simulink model "Converter_2"  (R2018a)
settings: Solver=ode45  StartTime=0.0  StopTime=3  FixedStep=Ts  RelTol=1e-3
InitFcn:
  | load('initial_C2.mat')
  | Ts=5e-4;
  | Ts_Power=Ts;
  | Ts_Control=Ts;
  | 
  | 
  | P_order = 0.9; %refrence power
  | V_order = .9965; %refrence voltage
  | Q_order = 0.4;
  | w_order = 1;
  | 
  | step_P_order = 2; %Step p_order at 5 sec.
  | 
  | %% DROOP COFFEICIENT
  | Kpf = 5; % Kpf = 1/m.
  | n = .1;
  | 
  | 
  | Kp = 0.3; Ki =5; % inner loop
  | %Outer loop
  | Kpp =1; Kip =100;
  | Kpv =.5; Kiv =50;
  | %Kpv =0.40; Kiv =40;
  | 
  | Kp_PLL = 60; Ki_PLL = 1400; % PLL 13 Hz
  | 
  | 
  | Cs = 0.25; % Shunt capacitor in pu
  | 
  | 
  | 
  | wb=2*pi*60;
  | Sb=10e3;
  | Vb=260;
  | Vconv=260;
  | Zb=Vb^2/Sb;
  | 
  | X=0.15;
  | 
  | %% Tirp Transmision line
  | Tstep3=5; % trip line: Xg_start-->Xg_mid
  | Tstep2=7; % trip line: Xg_mid-->Xg_final
  | 
  | 
  | 
  | Xg_start=1.172; Xg_mid=1.73; Xg_final=1.174;
  | %Xg_start=0.765; Xg_mid=0.95; Xg_final=1.08;
  | 
  | 
  | Xgpu2=Xg_mid*Xg_final/(Xg_final-Xg_mid);
  | Xgpu3=Xg_start*(Xg_final*Xgpu2)/(Xg_final*Xgpu2-Xg_start*(Xg_final+Xgpu2));
  | 
  | %Line 1
  | Xgpu1=Xg_final;
  | Rgpu1=0.1*Xgpu1;%Rg=0.1*Xg;
  | Xg1=Xgpu1*Zb;
  | Lg1=Xg1/wb;   %H
  | Rg1=Rgpu1*Zb; %ohm
  | %Line 2
  | Rgpu2=0.1*Xgpu2;%Rg=0.1*Xg;
  | Xg2=Xgpu2*Zb;
  | Lg2=Xg2/wb;   %H
  | Rg2=Rgpu2*Zb; %ohm
  | %Line 3
  | Rgpu3=0.1*Xgpu3;%Rg=0.1*Xg;
  | Xg3=Xgpu3*Zb;
  | Lg3=Xg3/wb;   %H
  | Rg3=Rgpu3*Zb; %ohm
undefined symbols (not defined in the file or in its folder): DiscIntNeverNeededParam
libraries: powerlib x14, powerlib_meascontrol x5, simulink x3
Description:
  | Copyright 2008-2017 The MathWorks, Inc.
settings Model: Creator=MathWorks  LastModifiedBy=almut
settings DataIOCC: FinalStateName=Sup_PLL2a  InitialState=Sup_PLL2a  LimitDataPoints=on  LoadInitialState=on  SaveFormat=Array  SignalLoggingSaveFormat=ModelDataLogs
settings OptimizationCC: ExpressionDepthLimit=2147483647  EfficientMapNaN2IntZero=off  LifeSpan=inf
settings DebuggingCC: UnderspecifiedInitializationDetection=Classic  MergeDetectMultiDrivingBlocksExec=none  SolverPrmCheckMsg=warning  FcnCallInpInsideContextMsg=warning  StateNameClashWarn=warning  SFUnexpectedBacktrackingDiag=warning  SFNoUnconditionalDefaultTransitionDiag=warning  SFExecutionAtInitializationDiag=none
settings HardwareCC: ProdBitPerPointer=32  ProdBitPerSizeT=32  ProdBitPerPtrDiffT=32  ProdLargestAtomicFloat=None  ProdIntDivRoundTo=Undefined  ProdEndianess=Unspecified  ProdWordSize=32  ProdHWDeviceType=32-bit Generic  TargetBitPerPointer=64  TargetBitPerSizeT=64  TargetBitPerPtrDiffT=64  TargetLongLongMode=on  TargetIntDivRoundTo=Zero  TargetEndianess=LittleEndian  TargetWordSize=64  TargetHWDeviceType=MATLAB Host  ProdEqTarget=off
settings ModelReferenceCC: PropagateSignalLabelsOutOfModel=off
settings CodeAppCC: MaxIdLength=128  StateflowObjectComments=on
settings GRTTargetCC: TargetLangStandard=C89/C90 (ANSI)  CombineOutputUpdateFcns=off  GRTInterface=on
settings ConfigComp: CovMetricSettings=dw  CovHtmlReporting=on  CovSaveCumulativeToWorkspaceVar=on  CovSaveSingleToWorkspaceVar=on  CovExternalEMLEnable=off  CovSFcnEnable=off
settings SimscapeCC: SimscapeNormalizeSystem=off

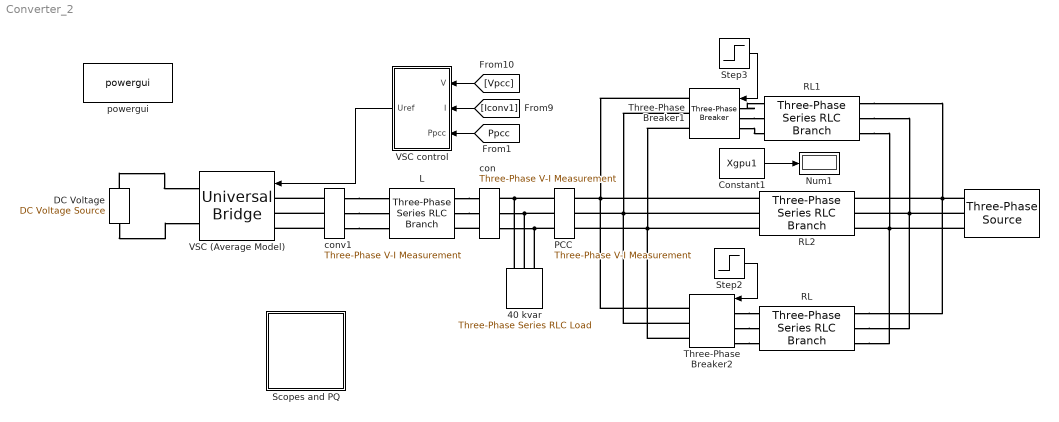
== system Converter_2 ==
  " " : powerlib/Electrical Sources/Three-Phase Source  InternalConnection=Yg  VoltagePhases=off  Voltage=260  PhaseAngle=0  Voltage_phases=[25e3 25e3 25e3]/sqrt(3)  PhaseAngles_phases=[0 -120 +120]  Frequency=60  NonIdealSource=off  SpecifyImpedance=on  Resistance=0.8929  Inductance=16.58e-3  ShortCircuitLevel=2500e6  BaseVoltage=120e3  XRratio=7  BusType=swing  Pref=0  Qref=0  Prefabc=[10e3, 10e3, 10e3]  Qrefabc=[0, 0, 0]  Qmin=-inf  Qmax=inf
  40 kvar : powerlib/Elements/Three-Phase Series RLC Load  LConnTagsString=A|B|C  Configuration=Y (grounded)  NominalVoltage=260  Vabc=[1e3 1e3 1e3]  Vabcp=[1e3 1e3 1e3]  NominalFrequency=60  UnbalancedPower=off  ActivePower=0  InductivePower=0  CapacitivePower=10e3*0.25  Pabc=[10e3 9e3 11e3]  QLabc=[100 90 110]  QCabc=[100 90 110]  Pabcp=[10e3 9e3 11e3]  QLabcp=[100 90 110]  QCabcp=[100 90 110]  Measurements=None  LoadType=constant Z
  Constant1 : Constant  Value=Xgpu1
  "DC Voltage " : powerlib/Electrical Sources/DC Voltage Source  Amplitude=500  Measurements=None
  L : powerlib/Elements/Three-Phase Series RLC Branch  LConnTagsString=A|B|C  RConnTagsString=A|B|C  BranchType=RL  Resistance=X/50*260^2/10e3  Inductance=X/(2*pi*60)*260^2/10e3  Capacitance=inf  Measurements=None
  Num1 : Display
  PCC : powerlib/Measurements/Three-Phase V-I Measurement  VoltageMeasurement=phase-to-ground  SetLabelV=on  LabelV=Vpcc  Vpu=on  VpuLL=off  CurrentMeasurement=yes  SetLabelI=on  LabelI=Ipcc  Ipu=on  Pbase=10e3  Vbase=260  OutputType=Magnitude  PhasorSimulation=off  PSBequivalent=0
  RL : powerlib/Elements/Three-Phase Series RLC Branch  LConnTagsString=A|B|C  RConnTagsString=A|B|C  BranchType=RL  Resistance=Rg2  Inductance=Lg2  Capacitance=[]  Measurements=None
  RL1 : powerlib/Elements/Three-Phase Series RLC Branch  LConnTagsString=A|B|C  RConnTagsString=A|B|C  BranchType=RL  Resistance=Rg3  Inductance=Lg3  Capacitance=[]  Measurements=None
  RL2 : powerlib/Elements/Three-Phase Series RLC Branch  LConnTagsString=A|B|C  RConnTagsString=A|B|C  BranchType=RL  Resistance=Rg1  Inductance=Lg1  Capacitance=[]  Measurements=None
  "Scopes and PQ " : Subsystem
  Step2 : Step  Time=Tstep2  Before=1  After=0  SampleTime=0
  Step3 : Step  Time=Tstep3  Before=1  After=0  SampleTime=0
  Three-Phase Breaker1 : powerlib/Elements/Three-Phase Breaker  InitialState=closed  SwitchA=on  SwitchB=on  SwitchC=on  SwitchTimes=[1 1000]  External=on  BreakerResistance=0.001  SnubberResistance=1e6  SnubberCapacitance=inf  Measurements=None
  Three-Phase Breaker2 : powerlib/Elements/Three-Phase Breaker  InitialState=closed  SwitchA=on  SwitchB=on  SwitchC=on  SwitchTimes=[1 1000]  External=on  BreakerResistance=0.001  SnubberResistance=1e6  SnubberCapacitance=inf  Measurements=None
  VSC (Average Model) : powerlib/Power Electronics/Universal Bridge  Arms=3  SnubberResistance=1e5  SnubberCapacitance=inf  Device=Average-model based VSC  Ron=1e-3  Lon=0  ForwardVoltages="[  0  0  ]"  ForwardVoltage=0  GTOparameters=[ 10e-6 , 20e-6 ]  IGBTparameters=[ 1e-6 , 2e-6 ]  Measurements=None  Measurements_2=None  converterType=Rectifier
  VSC control : Subsystem
  con : powerlib/Measurements/Three-Phase V-I Measurement  VoltageMeasurement=phase-to-ground  SetLabelV=on  LabelV=Vcon  Vpu=on  VpuLL=off  CurrentMeasurement=yes  SetLabelI=on  LabelI=Icon  Ipu=on  Pbase=10e3  Vbase=260  OutputType=Magnitude  PhasorSimulation=off  PSBequivalent=0
  conv1 : powerlib/Measurements/Three-Phase V-I Measurement  VoltageMeasurement=phase-to-ground  SetLabelV=on  LabelV=Vconv1  Vpu=on  VpuLL=off  CurrentMeasurement=yes  SetLabelI=on  LabelI=Iconv1  Ipu=on  Pbase=10e3  Vbase=260  OutputType=Magnitude  PhasorSimulation=off  PSBequivalent=0
  powergui : powerlib/powergui  Priority=1  SimulationMode=Discrete  SampleTime=Ts  frequency=60  Iterations=50  frequencyindice=0  Pbase=100e6  ErrMax=1e-4  UnitsV=kV  UnitsW=MW  buscounter=0  FunctionMessages=off  echomessages=off  EnableUseOfTLC=off  CurrentSourceSwitches=off  DisableSnubberDevices=off  DisableRonSwitches=off  DisableVfSwitches=off  DisplayEquations=off  SolverType=Tustin/Backward Euler (TBE)  Interpol=off  ExternalGateDelay=off  methode=off  Ts=100  x0status=blocks  SPID=off  SwTol=0  HookPort=off  RestoreLinks=warning  ResistiveCurrentMeasurement=off  Frange=[0:2:500]  Ylog=off  Xlog=on  ShowGrid=off  save=off  variable=ZData  structure=y  ZoomFFT=off  StartTime=2.5  cycles=30  DisplayStyle=2  fundamental=60  FreqAxis=off  MaxFrequency=100  frequencyindicesteady=1  RmsSteady=1  display=off
  wires:
  VSC control/1(Uref) -> VSC (Average Model)/1
  [Vpcc] -> VSC control/1(V)
  [Iconv1] -> VSC control/2(I)
  Step2/1 -> Three-Phase Breaker2/1
  Constant1/1 -> Num1/1
  Step3/1 -> Three-Phase Breaker1/1
  [Ppcc] -> VSC control/3(Ppcc)
  connections:
  con/LConn3 -- L/RConn3
  L/RConn1 -- con/LConn1
  L/RConn2 -- con/LConn2
  PCC/LConn1 -- 40 kvar/LConn1 -- con/RConn1
  con/RConn3 -- 40 kvar/LConn3 -- PCC/LConn3
  con/RConn2 -- 40 kvar/LConn2 -- PCC/LConn2
  conv1/RConn1 -- L/LConn1
  conv1/RConn3 -- L/LConn3
  conv1/RConn2 -- L/LConn2
  conv1/LConn1 -- VSC (Average Model)/LConn1
  conv1/LConn2 -- VSC (Average Model)/LConn2
  conv1/LConn3 -- VSC (Average Model)/LConn3
  "DC Voltage "/RConn1 -- VSC (Average Model)/RConn1
  "DC Voltage "/LConn1 -- VSC (Average Model)/RConn2
  Three-Phase Breaker2/LConn3 -- RL/RConn3
  Three-Phase Breaker2/LConn1 -- RL/RConn1
  Three-Phase Breaker2/LConn2 -- RL/RConn2
  Three-Phase Breaker1/LConn3 -- RL1/RConn3
  Three-Phase Breaker1/LConn2 -- RL1/RConn2
  Three-Phase Breaker1/LConn1 -- RL1/RConn1
  RL2/RConn1 -- Three-Phase Breaker2/RConn1 -- Three-Phase Breaker1/RConn1 -- PCC/RConn1
  RL2/RConn2 -- Three-Phase Breaker2/RConn2 -- Three-Phase Breaker1/RConn2 -- PCC/RConn2
  RL2/RConn3 -- Three-Phase Breaker2/RConn3 -- Three-Phase Breaker1/RConn3 -- PCC/RConn3
  " "/RConn1 -- RL/LConn1 -- RL1/LConn1 -- RL2/LConn1
  " "/RConn2 -- RL/LConn2 -- RL1/LConn2 -- RL2/LConn2
  " "/RConn3 -- RL/LConn3 -- RL1/LConn3 -- RL2/LConn3

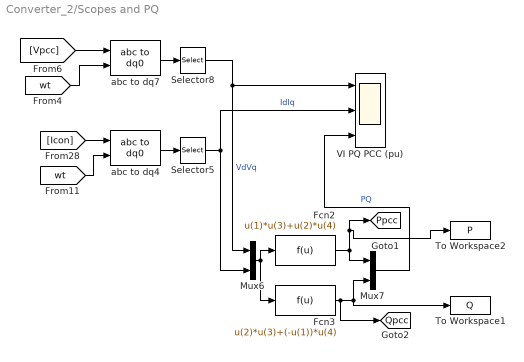
== system Converter_2/Scopes and PQ  ==
  Fcn2 : Fcn  Expr=u(1)*u(3)+u(2)*u(4)
  Fcn3 : Fcn  Expr=u(2)*u(3)+(-u(1))*u(4)
  Mux6 : Mux  Inputs=2
  Mux7 : Mux  Inputs=2
  Selector5 : Selector  InputPortWidth=3  IndexOptions=Index vector (dialog)  Indices=[1 2]  OutputSizes=1
  Selector8 : Selector  InputPortWidth=3  IndexOptions=Index vector (dialog)  Indices=[1 2]  OutputSizes=1
  To Workspace1 : ToWorkspace  VariableName=Q  SaveFormat=Timeseries  SampleTime=Ts
      settings: Save2DSignal=2-D array (concatenate along first dimension)
  To Workspace2 : ToWorkspace  VariableName=P  SaveFormat=Timeseries  SampleTime=Ts
      settings: Save2DSignal=2-D array (concatenate along first dimension)
  VI PQ PCC (pu) : Scope  NumInputPorts=3
  abc to dq4 : powerlib_meascontrol/Transformations/abc to dq0  Alignment=90 degrees behind phase A axis
  abc to dq7 : powerlib_meascontrol/Transformations/abc to dq0  Alignment=90 degrees behind phase A axis
  tag scope: Ppcc=global, Qpcc=global
  wires:
  abc to dq7/1 -> Selector8/1
  Mux6/1 -> Fcn3/1, Fcn2/1
  Mux7/1 -> VI PQ PCC (pu)/3  "PQ"
  [wt] -> abc to dq4/2
  Selector8/1 -> Mux6/1, VI PQ PCC (pu)/1  "VdVq"
  [Vpcc] -> abc to dq7/1
  Selector5/1 -> Mux6/2, VI PQ PCC (pu)/2  "IdIq"
  Fcn3/1 -> [Qpcc], To Workspace1/1, Mux7/2
  abc to dq4/1 -> Selector5/1
  [Icon] -> abc to dq4/1
  [wt] -> abc to dq7/2
  Fcn2/1 -> To Workspace2/1, [Ppcc], Mux7/1

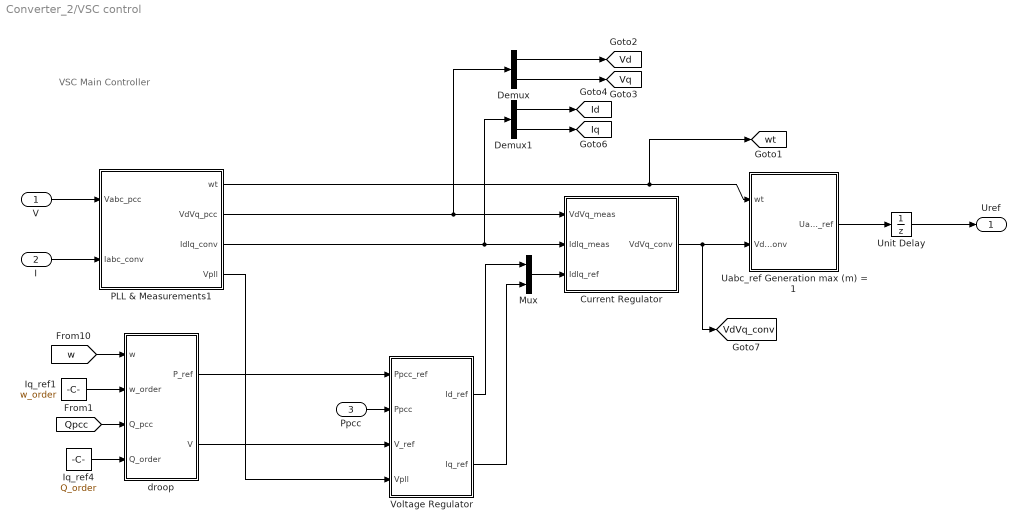
== system Converter_2/VSC control ==
  note: VSC Main Controller
  V : Inport  PortDimensions=3
  I : Inport  Port=2  PortDimensions=3
  Ppcc : Inport  Port=3  PortDimensions=1
  Current Regulator : Subsystem
  Demux : Demux  Outputs=2
  Demux1 : Demux  Outputs=2
  Iq_ref1 : Constant  Value=w_order
  Iq_ref4 : Constant  Value=Q_order
  Mux : Mux  Inputs=2
  PLL & Measurements1 : Subsystem
  Uabc_ref Generation max (m) = 1 : Subsystem
  Unit Delay : UnitDelay  SampleTime=Ts_Control
  Voltage Regulator : Subsystem
  droop : Subsystem
  Uref : Outport
  tag scope: Id=global, Iq=global, Vd=global, VdVq_conv=global, Vq=global, wt=global
  wires:
  Demux/2 -> [Vq]
  Demux/1 -> [Vd]
  Unit Delay/1 -> Uref/1
  Demux1/1 -> [Id]
  Mux/1 -> Current Regulator/3(IdIq_ref)
  PLL & Measurements1/1(wt) -> [wt], Uabc_ref Generation max (m) = 1/1(wt)
  Current Regulator/1(VdVq_conv) -> [VdVq_conv], Uabc_ref Generation max (m) = 1/2(VdVq_conv)
  Uabc_ref Generation max (m) = 1/1(Uabc_ref) -> Unit Delay/1
  Demux1/2 -> [Iq]
  I/1 -> PLL & Measurements1/2(Iabc_conv)
  V/1 -> PLL & Measurements1/1(Vabc_pcc)
  PLL & Measurements1/3(IdIq_conv) -> Demux1/1, Current Regulator/2(IdIq_meas)
  PLL & Measurements1/2(VdVq_pcc) -> Demux/1, Current Regulator/1(VdVq_meas)
  Voltage Regulator/1(Id_ref) -> Mux/1
  Voltage Regulator/2(Iq_ref) -> Mux/2
  Ppcc/1 -> Voltage Regulator/2(Ppcc)
  PLL & Measurements1/4(Vpll) -> Voltage Regulator/4(Vpll)
  droop/1(P_ref) -> Voltage Regulator/1(Ppcc_ref)
  Iq_ref4/1 -> droop/4(Q_order)
  [w] -> droop/1(w)
  droop/2(V) -> Voltage Regulator/3(V_ref)
  [Qpcc] -> droop/3(Q_pcc)
  Iq_ref1/1 -> droop/2(w_order)

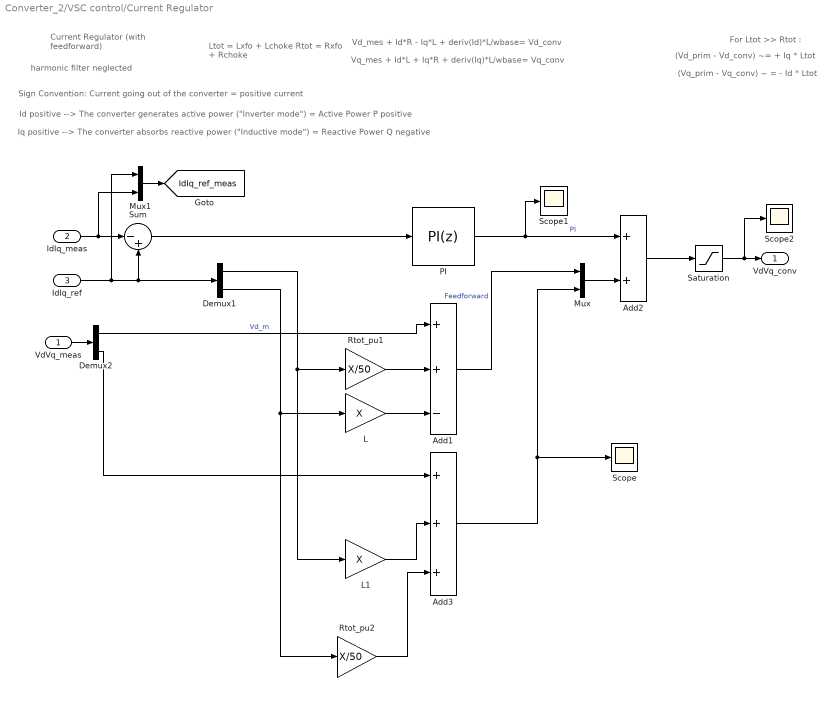
== system Converter_2/VSC control/Current Regulator ==
  note: For Ltot >> Rtot :
  note: (Vq_prim - Vq_conv) ~ = - Id * Ltot
  note: (Vd_prim - Vd_conv) ~= + Iq * Ltot
  note: Ltot = Lxfo + Lchoke
      | Rtot = Rxfo + Rchoke
  note: Id positive --> The converter generates active power ("Inverter mode") = Active Power P positive
  note: Iq positive --> The converter absorbs reactive power ("Inductive mode") = Reactive Power Q negative
  note: Sign Convention: Current going out of the converter = positive current
  note: Current Regulator
      | (with feedforward)
  note: Vq_mes + Id*L + Iq*R + deriv(Iq)*L/wbase= Vq_conv
  note: Vd_mes + Id*R - Iq*L + deriv(Id)*L/wbase= Vd_conv
  note: harmonic filter neglected
  VdVq_meas : Inport  PortDimensions=2
  IdIq_meas : Inport  Port=2  PortDimensions=2
  IdIq_ref : Inport  Port=3  PortDimensions=2
  Add1 : Sum  Inputs=++-
  Add2 : Sum
  Add3 : Sum  Inputs=+++
  Demux1 : Demux  Outputs=2
  Demux2 : Demux  Outputs=2
  L : Gain  Gain=X  SaturateOnIntegerOverflow=on  OutDataTypeStr=Inherit: Same as input  ParamDataTypeStr=Inherit: Same as input
  L1 : Gain  Gain=X  SaturateOnIntegerOverflow=on  OutDataTypeStr=Inherit: Same as input  ParamDataTypeStr=Inherit: Same as input
  Mux : Mux  Inputs=2
  Mux1 : Mux  Inputs=2
  PI : simulink/Continuous/PID Controller  Controller=PI  TimeDomain=Discrete-time  SampleTime=Ts  IntegratorMethod=Forward Euler  FilterMethod=Forward Euler  Form=Parallel  UseFilter=on  ControllerParametersSource=internal  P=Kp  I=Ki  D=0  N=100  InitialConditionSource=internal  InitialConditionForIntegrator=0  InitialConditionForFilter=0  ExternalReset=none  LimitOutput=on  UpperSaturationLimit=2  LowerSaturationLimit=-2  LinearizeAsGain=off  AntiWindupMode=none  Kb=1  TrackingMode=off  Kt=1  PParamMin=[]  PParamMax=[]  IParamMin=[]  IParamMax=[]  DParamMin=[]  DParamMax=[]  NParamMin=[]  NParamMax=[]  KbParamMin=[]  KbParamMax=[]  KtParamMin=[]  KtParamMax=[]  POutMin=[]  POutMax=[]  IOutMin=[]  IOutMax=[]  DOutMin=[]  DOutMax=[]  NOutMin=[]  NOutMax=[]  KbOutMin=[]  KbOutMax=[]  KtOutMin=[]  KtOutMax=[]  IntegratorOutMin=[]  IntegratorOutMax=[]  FilterOutMin=[]  FilterOutMax=[]  SumOutMin=[]  SumOutMax=[]  SumI1OutMin=[]  SumI1OutMax=[]  SumI2OutMin=[]  SumI2OutMax=[]  SumI3OutMin=[]  SumI3OutMax=[]  SumDOutMin=[]  SumDOutMax=[]  SaturationOutMin=[]  SaturationOutMax=[]  IntegratorContinuousStateAttributes=''  IntegratorStateMustResolveToSignalObject=off  IntegratorRTWStateStorageClass=Auto  FilterContinuousStateAttributes=''  FilterStateMustResolveToSignalObject=off  FilterRTWStateStorageClass=Auto  DifferentiatorICPrevScaledInput=0  DifferentiatorOutMin=[]  DifferentiatorOutMax=[]  FilterDiffOutCoefMin=[]  FilterDiffOutCoefMax=[]  SumDenOutMin=[]  SumDenOutMax=[]  SumNumOutMin=[]  SumNumOutMax=[]  ReciprocalOutMin=[]  ReciprocalOutMax=[]  DivideOutMin=[]  DivideOutMax=[]  TunerSelectOption=Transfer Function Based (PID Tuner App)
  Rtot_pu1 : Gain  Gain=X/50  SaturateOnIntegerOverflow=on  OutDataTypeStr=Inherit: Same as input  ParamDataTypeStr=Inherit: Same as input
  Rtot_pu2 : Gain  Gain=X/50  SaturateOnIntegerOverflow=on  OutDataTypeStr=Inherit: Same as input  ParamDataTypeStr=Inherit: Same as input
  Saturation : Saturate  UpperLimit=2  LowerLimit=-2
  Scope : Scope
  Scope1 : Scope
  Scope2 : Scope
  Sum : Sum  Inputs=|-+
  VdVq_conv : Outport
  tag scope: IdIq_ref_meas=global
  wires:
  Add1/1 -> Mux/1  "Feedforward"
  Demux1/2 -> Rtot_pu2/1, L/1
  Demux1/1 -> Rtot_pu1/1, L1/1
  VdVq_meas/1 -> Demux2/1
  Saturation/1 -> Scope2/1, VdVq_conv/1
  Add2/1 -> Saturation/1
  Mux/1 -> Add2/2
  Mux1/1 -> [IdIq_ref_meas]
  Add3/1 -> Scope/1, Mux/2
  Sum/1 -> PI/1
  PI/1 -> Scope1/1, Add2/1  "PI"
  Demux2/1 -> Add1/1  "Vd_m"
  L1/1 -> Add3/2
  IdIq_meas/1 -> Sum/1, Mux1/2
  IdIq_ref/1 -> Demux1/1, Sum/2, Mux1/1
  Demux2/2 -> Add3/1
  L/1 -> Add1/3
  Rtot_pu1/1 -> Add1/2
  Rtot_pu2/1 -> Add3/3

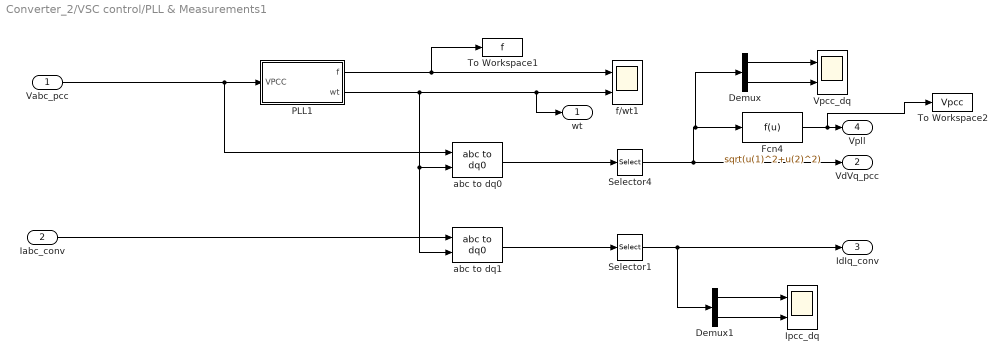
== system Converter_2/VSC control/PLL & Measurements1 ==
  Vabc_pcc : Inport
  Iabc_conv : Inport  Port=2
  Demux : Demux  Outputs=2
  Demux1 : Demux  Outputs=2
  Fcn4 : Fcn  Expr=sqrt(u(1)^2+u(2)^2)
  Ipcc_dq : Scope  NumInputPorts=2
  PLL1 : Subsystem
  Selector1 : Selector  InputPortWidth=3  IndexOptions=Index vector (dialog)  Indices=[1 2]  OutputSizes=1
  Selector4 : Selector  InputPortWidth=3  IndexOptions=Index vector (dialog)  Indices=[1 2]  OutputSizes=1
  To Workspace1 : ToWorkspace  VariableName=f  SaveFormat=Timeseries  SampleTime=Ts
      settings: Save2DSignal=2-D array (concatenate along first dimension)
  To Workspace2 : ToWorkspace  VariableName=Vpcc  SaveFormat=Timeseries  SampleTime=Ts
      settings: Save2DSignal=2-D array (concatenate along first dimension)
  Vpcc_dq : Scope  NumInputPorts=2
  abc to dq0 : powerlib_meascontrol/Transformations/abc to dq0  Alignment=90 degrees behind phase A axis
  abc to dq1 : powerlib_meascontrol/Transformations/abc to dq0  Alignment=90 degrees behind phase A axis
  f/wt1 : Scope  NumInputPorts=2
  wt : Outport
  VdVq_pcc : Outport  Port=2
  IdIq_conv : Outport  Port=3
  Vpll : Outport  Port=4
  wires:
  PLL1/2(wt) -> abc to dq0/2, abc to dq1/2, wt/1, f/wt1/2
  Vabc_pcc/1 -> PLL1/1(VPCC), abc to dq0/1
  Iabc_conv/1 -> abc to dq1/1
  abc to dq0/1 -> Selector4/1
  abc to dq1/1 -> Selector1/1
  Selector1/1 -> Demux1/1, IdIq_conv/1
  Demux/1 -> Vpcc_dq/1
  Demux/2 -> Vpcc_dq/2
  Demux1/1 -> Ipcc_dq/1
  Demux1/2 -> Ipcc_dq/2
  Selector4/1 -> Demux/1, Fcn4/1, VdVq_pcc/1
  Fcn4/1 -> To Workspace2/1, Vpll/1
  PLL1/1(f) -> To Workspace1/1, f/wt1/1

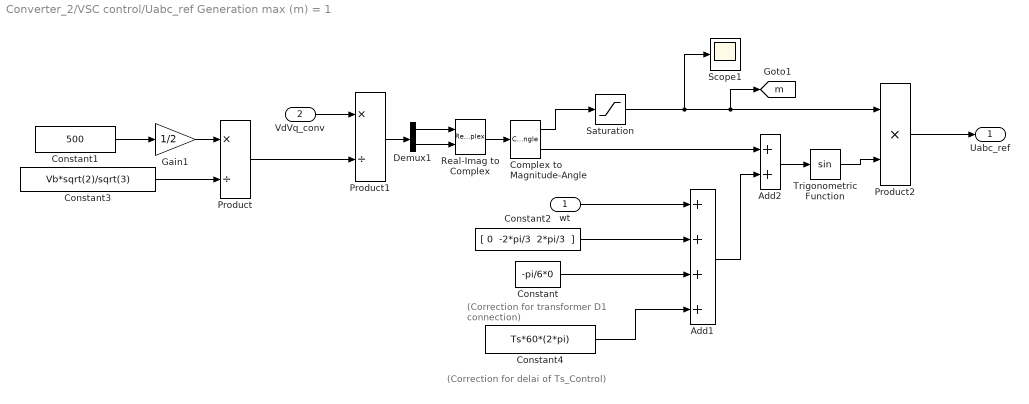
== system Converter_2/VSC control/Uabc_ref Generation max (m) = 1 ==
  note: (Correction for delai of Ts_Control)
  note: (Correction for transformer
      |  D1 connection)
  wt : Inport
  VdVq_conv : Inport  Port=2
  Add1 : Sum  Inputs=++++
  Add2 : Sum
  Complex to Magnitude-Angle : ComplexToMagnitudeAngle
  Constant : Constant  Value=-pi/6*0
  Constant1 : Constant  Value=500
  Constant2 : Constant  Value="[ 0  -2*pi/3  2*pi/3  ]"
  Constant3 : Constant  Value=Vb*sqrt(2)/sqrt(3)
  Constant4 : Constant  Value=Ts*60*(2*pi)
  Demux1 : Demux  Outputs=2
  Gain1 : Gain  Gain=1/2
  Product : Product  Inputs=*/  RndMeth=Zero
  Product1 : Product  Inputs=*/  RndMeth=Zero
  Product2 : Product  Inputs=**  RndMeth=Zero
  Real-Imag to Complex : RealImagToComplex
  Saturation : Saturate  UpperLimit=1  LowerLimit=0
  Scope1 : Scope
  Trigonometric Function : Trigonometry
  Uabc_ref : Outport
  tag scope: m=global
  wires:
  Constant4/1 -> Add1/4
  wt/1 -> Add1/1
  Product2/1 -> Uabc_ref/1
  Trigonometric Function/1 -> Product2/2
  Add2/1 -> Trigonometric Function/1
  Add1/1 -> Add2/2
  Complex to Magnitude-Angle/2 -> Add2/1
  Product/1 -> Product1/2
  Constant3/1 -> Product/2
  Constant/1 -> Add1/3
  Constant2/1 -> Add1/2
  Demux1/2 -> Real-Imag to Complex/2
  Demux1/1 -> Real-Imag to Complex/1
  Real-Imag to Complex/1 -> Complex to Magnitude-Angle/1
  Gain1/1 -> Product/1
  Product1/1 -> Demux1/1
  VdVq_conv/1 -> Product1/1
  Constant1/1 -> Gain1/1
  Complex to Magnitude-Angle/1 -> Saturation/1
  Saturation/1 -> Scope1/1, Product2/1, [m]

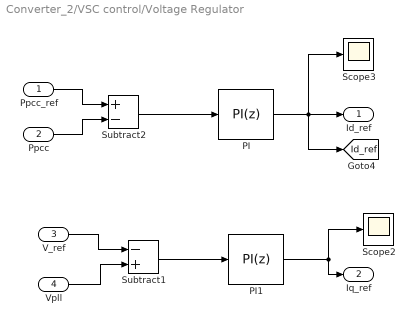
== system Converter_2/VSC control/Voltage Regulator ==
  Ppcc_ref : Inport  PortDimensions=1
  Ppcc : Inport  Port=2  PortDimensions=1
  V_ref : Inport  Port=3  PortDimensions=1
  Vpll : Inport  Port=4  PortDimensions=1
  PI : simulink/Continuous/PID Controller  Controller=PI  TimeDomain=Discrete-time  SampleTime=Ts  IntegratorMethod=Trapezoidal  FilterMethod=Forward Euler  Form=Parallel  UseFilter=on  ControllerParametersSource=internal  P=Kpp  I=Kip  D=0  N=100  InitialConditionSource=internal  InitialConditionForIntegrator=0  InitialConditionForFilter=0  ExternalReset=none  LimitOutput=on  UpperSaturationLimit=1.5  LowerSaturationLimit=-1.5  LinearizeAsGain=off  AntiWindupMode=none  Kb=1  TrackingMode=off  Kt=1  PParamMin=[]  PParamMax=[]  IParamMin=[]  IParamMax=[]  DParamMin=[]  DParamMax=[]  NParamMin=[]  NParamMax=[]  KbParamMin=[]  KbParamMax=[]  KtParamMin=[]  KtParamMax=[]  POutMin=[]  POutMax=[]  IOutMin=[]  IOutMax=[]  DOutMin=[]  DOutMax=[]  NOutMin=[]  NOutMax=[]  KbOutMin=[]  KbOutMax=[]  KtOutMin=[]  KtOutMax=[]  IntegratorOutMin=[]  IntegratorOutMax=[]  FilterOutMin=[]  FilterOutMax=[]  SumOutMin=[]  SumOutMax=[]  SumI1OutMin=[]  SumI1OutMax=[]  SumI2OutMin=[]  SumI2OutMax=[]  SumI3OutMin=[]  SumI3OutMax=[]  SumDOutMin=[]  SumDOutMax=[]  SaturationOutMin=[]  SaturationOutMax=[]  IntegratorContinuousStateAttributes=''  IntegratorStateMustResolveToSignalObject=off  IntegratorRTWStateStorageClass=Auto  FilterContinuousStateAttributes=''  FilterStateMustResolveToSignalObject=off  FilterRTWStateStorageClass=Auto  DifferentiatorICPrevScaledInput=0  DifferentiatorOutMin=[]  DifferentiatorOutMax=[]  FilterDiffOutCoefMin=[]  FilterDiffOutCoefMax=[]  SumDenOutMin=[]  SumDenOutMax=[]  SumNumOutMin=[]  SumNumOutMax=[]  ReciprocalOutMin=[]  ReciprocalOutMax=[]  DivideOutMin=[]  DivideOutMax=[]  TunerSelectOption=Transfer Function Based (PID Tuner App)
  PI1 : simulink/Continuous/PID Controller  Controller=PI  TimeDomain=Discrete-time  SampleTime=Ts  IntegratorMethod=Trapezoidal  FilterMethod=Forward Euler  Form=Parallel  UseFilter=on  ControllerParametersSource=internal  P=Kpv  I=Kiv  D=0  N=100  InitialConditionSource=internal  InitialConditionForIntegrator=0  InitialConditionForFilter=0  ExternalReset=none  LimitOutput=on  UpperSaturationLimit=1.5  LowerSaturationLimit=-1.5  LinearizeAsGain=off  AntiWindupMode=none  Kb=1  TrackingMode=off  Kt=1  PParamMin=[]  PParamMax=[]  IParamMin=[]  IParamMax=[]  DParamMin=[]  DParamMax=[]  NParamMin=[]  NParamMax=[]  KbParamMin=[]  KbParamMax=[]  KtParamMin=[]  KtParamMax=[]  POutMin=[]  POutMax=[]  IOutMin=[]  IOutMax=[]  DOutMin=[]  DOutMax=[]  NOutMin=[]  NOutMax=[]  KbOutMin=[]  KbOutMax=[]  KtOutMin=[]  KtOutMax=[]  IntegratorOutMin=[]  IntegratorOutMax=[]  FilterOutMin=[]  FilterOutMax=[]  SumOutMin=[]  SumOutMax=[]  SumI1OutMin=[]  SumI1OutMax=[]  SumI2OutMin=[]  SumI2OutMax=[]  SumI3OutMin=[]  SumI3OutMax=[]  SumDOutMin=[]  SumDOutMax=[]  SaturationOutMin=[]  SaturationOutMax=[]  IntegratorContinuousStateAttributes=''  IntegratorStateMustResolveToSignalObject=off  IntegratorRTWStateStorageClass=Auto  FilterContinuousStateAttributes=''  FilterStateMustResolveToSignalObject=off  FilterRTWStateStorageClass=Auto  DifferentiatorICPrevScaledInput=0  DifferentiatorOutMin=[]  DifferentiatorOutMax=[]  FilterDiffOutCoefMin=[]  FilterDiffOutCoefMax=[]  SumDenOutMin=[]  SumDenOutMax=[]  SumNumOutMin=[]  SumNumOutMax=[]  ReciprocalOutMin=[]  ReciprocalOutMax=[]  DivideOutMin=[]  DivideOutMax=[]  TunerSelectOption=Transfer Function Based (PID Tuner App)
  Scope2 : Scope
  Scope3 : Scope
  Subtract1 : Sum  Inputs=-+
  Subtract2 : Sum  Inputs=+-
  Id_ref : Outport  SampleTime=Ts  InitialOutput=0
  Iq_ref : Outport  Port=2  SampleTime=Ts  InitialOutput=0
  tag scope: Id_ref=global
  wires:
  PI/1 -> Scope3/1, Id_ref/1, [Id_ref]
  PI1/1 -> Iq_ref/1, Scope2/1
  Subtract2/1 -> PI/1
  Subtract1/1 -> PI1/1
  Ppcc_ref/1 -> Subtract2/1
  Ppcc/1 -> Subtract2/2
  Vpll/1 -> Subtract1/2
  V_ref/1 -> Subtract1/1

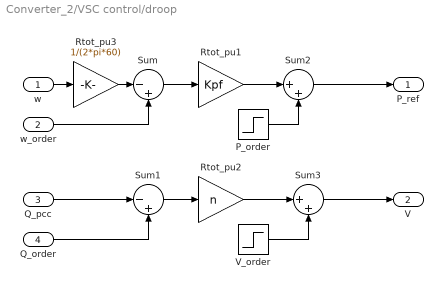
== system Converter_2/VSC control/droop ==
  w : Inport
  w_order : Inport  Port=2
  Q_pcc : Inport  Port=3
  Q_order : Inport  Port=4
  P_order : Step  Time=step_P_order  Before=P_order  After=P_order+0.01  SampleTime=0
  Rtot_pu1 : Gain  Gain=Kpf  SaturateOnIntegerOverflow=on  OutDataTypeStr=Inherit: Same as input  ParamDataTypeStr=Inherit: Same as input
  Rtot_pu2 : Gain  Gain=n  SaturateOnIntegerOverflow=on  OutDataTypeStr=Inherit: Same as input  ParamDataTypeStr=Inherit: Same as input
  Rtot_pu3 : Gain  Gain=1/(2*pi*60)  SaturateOnIntegerOverflow=on  OutDataTypeStr=Inherit: Same as input  ParamDataTypeStr=Inherit: Same as input
  Sum : Sum  Inputs=|-+
  Sum1 : Sum  Inputs=|-+
  Sum2 : Sum  Inputs=|++
  Sum3 : Sum  Inputs=|++
  V_order : Step  Time=33  Before=V_order  After=1.06  SampleTime=0
  P_ref : Outport
  V : Outport  Port=2
  wires:
  V_order/1 -> Sum3/2
  Sum/1 -> Rtot_pu1/1
  Sum1/1 -> Rtot_pu2/1
  Sum2/1 -> P_ref/1
  Rtot_pu2/1 -> Sum3/1
  Rtot_pu1/1 -> Sum2/1
  P_order/1 -> Sum2/2
  Sum3/1 -> V/1
  Q_order/1 -> Sum1/2
  w_order/1 -> Sum/2
  Q_pcc/1 -> Sum1/1
  w/1 -> Rtot_pu3/1
  Rtot_pu3/1 -> Sum/1

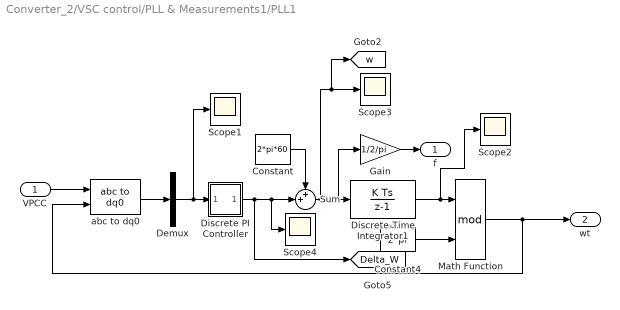
== system Converter_2/VSC control/PLL & Measurements1/PLL1 ==
  VPCC : Inport
  Constant : Constant  Value=2*pi*60
  Constant4 : Constant  Value=2*pi  SampleTime=Ts
  Demux : Demux  Outputs=3
  Discrete PI Controller : Subsystem  DialogController=POWERSYS.PowerSysDialog  mask(Discrete PI Controller){Kp=Kp_PLL, Ki=Ki_PLL, Par_Limits=[1 -1]*inf, Init=0, Ts=Ts}
      mask prompts: Kp "Proportional gain (Kp):"; Ki "Integral gain (Ki):"; Par_Limits "Output limits: [ Upper   Lower ]"; Init "Output initial value:"; Ts "Sample time:"
      mask help: This block implements a discrete PI controller.
      mask init:
      | UpperLimit=Par_Limits(1);
      | LowerLimit=Par_Limits(2);
      | power_initmask();
      mask Help: This block is part of a subset of blocks in the Extras library that does not have documentation associated with it, other than the block mask description.
      mask Display: disp('PI');
  Discrete-Time Integrator1 : DiscreteIntegrator  gainval=1  SampleTime=Ts  LimitOutput=on  ICPrevOutput=DiscIntNeverNeededParam  ICPrevScaledInput=DiscIntNeverNeededParam
  Gain : Gain  Gain=1/2/pi
  Math Function : Math  Operator=mod  SaturateOnIntegerOverflow=on
  Scope{1..4} (4 alike) : Scope
  Sum : Sum  Inputs=++|
  abc to dq0 : powerlib_meascontrol/Transformations/abc to dq0  Alignment=90 degrees behind phase A axis
  f : Outport
  wt : Outport  Port=2
  tag scope: Delta_W=global, w=global
  wires:
  VPCC/1 -> abc to dq0/1
  abc to dq0/1 -> Demux/1
  Demux/2 -> Discrete PI Controller/1(Error), Scope1/1
  Sum/1 -> [w], Scope3/1, Gain/1, Discrete-Time Integrator1/1
  Constant/1 -> Sum/1
  Gain/1 -> f/1
  Constant4/1 -> Math Function/2
  Discrete-Time Integrator1/1 -> Scope2/1, Math Function/1
  Math Function/1 -> abc to dq0/2, wt/1
  Discrete PI Controller/1(Out) -> [Delta_W], Scope4/1, Sum/2

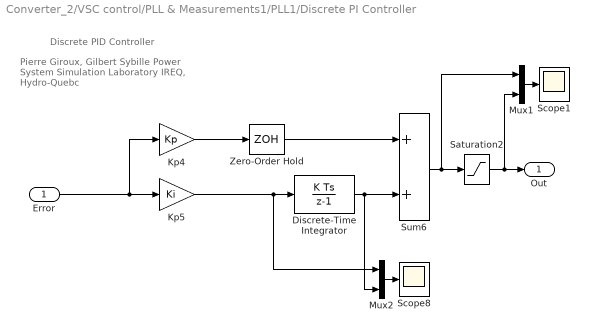
== system Converter_2/VSC control/PLL & Measurements1/PLL1/Discrete PI Controller ==
  note: Discrete PID Controller
  note: Pierre Giroux, Gilbert Sybille
      | Power System Simulation Laboratory
      | IREQ, Hydro-Quebc
  Error : Inport  SampleTime=Ts
  Discrete-Time Integrator : DiscreteIntegrator  InitialCondition=Init  SampleTime=Ts  LimitOutput=on  UpperSaturationLimit=UpperLimit  LowerSaturationLimit=LowerLimit  ICPrevOutput=DiscIntNeverNeededParam  ICPrevScaledInput=DiscIntNeverNeededParam
  Kp4 : Gain  Gain=Kp  SampleTime=Ts  SaturateOnIntegerOverflow=on  OutDataTypeStr=Inherit: Same as input  ParamDataTypeStr=Inherit: Same as input
  Kp5 : Gain  Gain=Ki  SampleTime=Ts  SaturateOnIntegerOverflow=on  OutDataTypeStr=Inherit: Same as input  ParamDataTypeStr=Inherit: Same as input
  Mux1 : Mux  Inputs=2
  Mux2 : Mux  Inputs=2
  Saturation2 : Saturate  UpperLimit=UpperLimit  LowerLimit=LowerLimit  SampleTime=Ts
  Scope1 : Scope
  Scope8 : Scope
  Sum6 : Sum  SampleTime=Ts  SaturateOnIntegerOverflow=on  InputSameDT=on  OutDataTypeStr=Inherit: Same as first input
  Zero-Order Hold : ZeroOrderHold  SampleTime=Ts
  Out : Outport  SampleTime=Ts  InitialOutput=0
  wires:
  Zero-Order Hold/1 -> Sum6/1
  Saturation2/1 -> Mux1/2, Out/1
  Discrete-Time Integrator/1 -> Mux2/2, Sum6/2
  Kp4/1 -> Zero-Order Hold/1
  Kp5/1 -> Mux2/1, Discrete-Time Integrator/1
  Sum6/1 -> Mux1/1, Saturation2/1
  Error/1 -> Kp5/1, Kp4/1
  Mux2/1 -> Scope8/1
  Mux1/1 -> Scope1/1
